simulink model "t1simu"  (R2023b)
settings: Solver=VariableStepAuto  StartTime=0.0  StopTime=10.0  RelTol=1e-3  EnableMultiTasking=on
settings Model: Creator=Admin  LastModifiedBy=danish
settings SolverCC: AlgebraicLoopSolver=TrustRegion
settings DataIOCC: ReturnWorkspaceOutputs=off
settings OptimizationCC: LifeSpan=inf
settings DebuggingCC: UnconnectedInputMsg=warning  UnconnectedOutputMsg=warning  UnconnectedLineMsg=warning  SFUnexpectedBacktrackingDiag=warning  SFNoUnconditionalDefaultTransitionDiag=warning  ArithmeticOperatorsInVariantConditions=warning
settings ModelReferenceCC: EnableRefExpFcnMdlSchedulingChecks=on
settings SFSimCC: SimUseLocalCustomCode=off  CustomCodeUndefinedFunction=UseInterfaceOnly
settings RTWCC: RTWUseLocalCustomCode=off
settings CodeAppCC: StateflowObjectComments=on
settings GRTTargetCC: TargetLangStandard=C89/C90 (ANSI)
settings ConfigComp: CovMetricSettings=dw  CovSaveCumulativeToWorkspaceVar=on  CovSaveSingleToWorkspaceVar=on  CovExternalEMLEnable=off

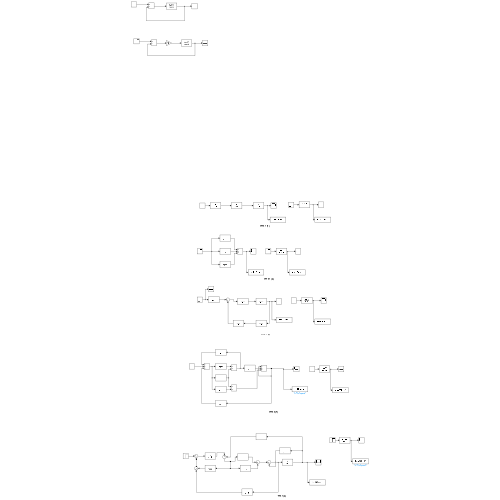
[thumbnail: Simulink's stored preview of the top-level diagram]
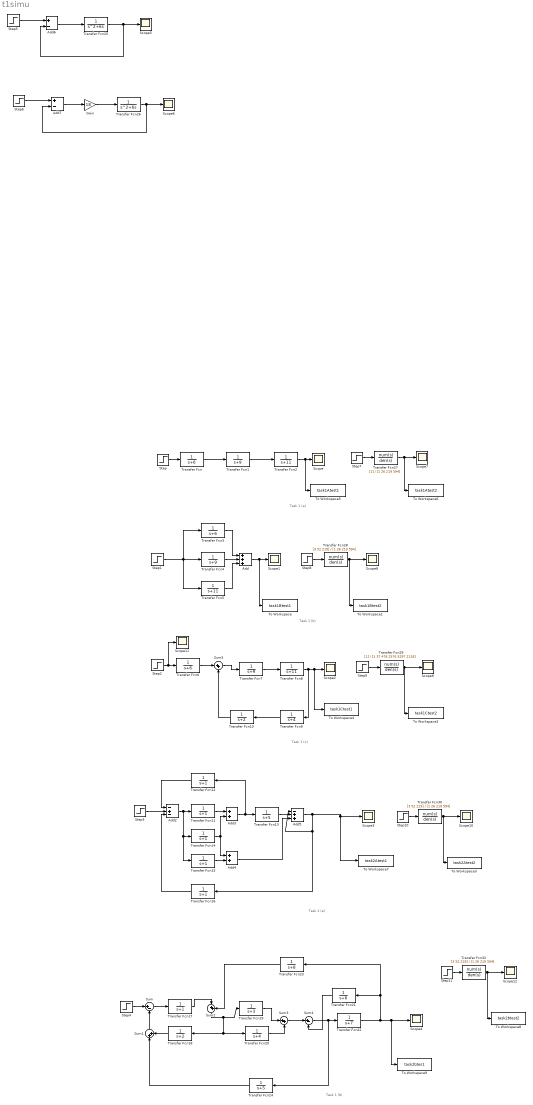
== system t1simu ==
  note: Task 1 (a)
  note: Task 1 (b)
  note: Task 1 (c)
  note: Task 2 (a)
  note: Task 1 (b)
  Add : Sum  Inputs=+++
  Add2 : Sum  Inputs=-+-
  Add3 : Sum
  Add4 : Sum
  Add5 : Sum  Inputs=-++
  Add6 : Sum  Inputs=+-
  Add7 : Sum  Inputs=+-
  Gain : Gain  Gain=18
  Scope{,1..12} (13 alike) : Scope
  Step{,1..11} (12 alike) : Step  Time=0  SampleTime=0
  Sum : Sum  Inputs=|+-
  Sum{1..3,5} (4 alike) : Sum  Inputs=|++
  Sum4 : Sum  Inputs=|+-
  To Workspace : ToWorkspace  VariableName=task1Btest1  SaveFormat=Timeseries  SampleTime=-1
  To Workspace1 : ToWorkspace  VariableName=task1Btest2  SaveFormat=Timeseries  SampleTime=-1
  To Workspace2 : ToWorkspace  VariableName=task1Ctest2  SaveFormat=Timeseries  SampleTime=-1
  To Workspace3 : ToWorkspace  VariableName=task2Atest2  SaveFormat=Timeseries  SampleTime=-1
  To Workspace4 : ToWorkspace  VariableName=task1Ctest1  SaveFormat=Timeseries  SampleTime=-1
  To Workspace5 : ToWorkspace  VariableName=task1Atest1  SaveFormat=Timeseries  SampleTime=-1
  To Workspace6 : ToWorkspace  VariableName=task1Atest2  SaveFormat=Timeseries  SampleTime=-1
  To Workspace7 : ToWorkspace  VariableName=task2Atest1  SaveFormat=Timeseries  SampleTime=-1
  To Workspace8 : ToWorkspace  VariableName=task2btest2  SaveFormat=Timeseries  SampleTime=-1
  To Workspace9 : ToWorkspace  VariableName=task2btes1  SaveFormat=Timeseries  SampleTime=-1
  Transfer Fcn{,3,6,21} (4 alike) : TransferFcn  Denominator=[1 6]
  Transfer Fcn1 : TransferFcn  Denominator=[1 9]
  Transfer Fcn10 : TransferFcn  Denominator=[1 2]
  Transfer Fcn{11..12,14..17} (6 alike) : TransferFcn  Denominator=[1 1]
  Transfer Fcn13 : TransferFcn  Denominator=[1 5]
  Transfer Fcn18 : TransferFcn  Denominator=[1 2]
  Transfer Fcn19 : TransferFcn  Denominator=[1 3]
  Transfer Fcn2 : TransferFcn  Denominator=[1 11]
  Transfer Fcn20 : TransferFcn  Denominator=[1 4]
  Transfer Fcn22 : TransferFcn  Denominator=[1 7]
  Transfer Fcn23 : TransferFcn  Denominator=[1 8]
  Transfer Fcn24 : TransferFcn  Denominator=[1 5]
  Transfer Fcn25 : TransferFcn  Denominator=[1 6 0]
  Transfer Fcn26 : TransferFcn  Denominator=[1 6 0]
  Transfer Fcn27 : TransferFcn  Denominator=[1 26 219 594]
  Transfer Fcn28 : TransferFcn  Numerator=[3 52 219]  Denominator=[1 26 219 594]
  Transfer Fcn29 : TransferFcn  Denominator=[1 37 478 2576 5297 2118]
  Transfer Fcn30 : TransferFcn  Numerator=[3 52 219]  Denominator=[1 26 219 594]
  Transfer Fcn32 : TransferFcn  Numerator=[3 52 219]  Denominator=[1 26 219 594]
  Transfer Fcn4 : TransferFcn  Denominator=[1 9]
  Transfer Fcn5 : TransferFcn  Denominator=[1 11]
  Transfer Fcn7 : TransferFcn  Denominator=[1 9]
  Transfer Fcn8 : TransferFcn  Denominator=[1 11]
  Transfer Fcn9 : TransferFcn  Denominator=[1 4]
  wires:
  Transfer Fcn1/1 -> Transfer Fcn2/1
  Transfer Fcn/1 -> Transfer Fcn1/1
  Step/1 -> Transfer Fcn/1
  Step1/1 -> Transfer Fcn3/1, Transfer Fcn5/1, Transfer Fcn4/1
  Transfer Fcn4/1 -> Add/2
  Transfer Fcn3/1 -> Add/1
  Transfer Fcn5/1 -> Add/3
  Add/1 -> To Workspace/1, Scope1/1
  Transfer Fcn6/1 -> Sum5/1
  Sum5/1 -> Transfer Fcn7/1
  Transfer Fcn7/1 -> Transfer Fcn8/1
  Transfer Fcn10/1 -> Sum5/2
  Transfer Fcn12/1 -> Add2/1
  Step3/1 -> Add2/2
  Transfer Fcn11/1 -> Add3/1
  Add2/1 -> Transfer Fcn15/1, Transfer Fcn14/1, Transfer Fcn11/1
  Add3/1 -> Transfer Fcn12/1, Transfer Fcn13/1
  Transfer Fcn14/1 -> Add4/1, Add3/2
  Transfer Fcn15/1 -> Add4/2
  Transfer Fcn13/1 -> Add5/2
  Transfer Fcn16/1 -> Add2/3
  Add4/1 -> Add5/3
  Step4/1 -> Sum/1
  Sum/1 -> Transfer Fcn17/1
  Sum1/1 -> Sum/2
  Transfer Fcn17/1 -> Sum2/1
  Transfer Fcn18/1 -> Sum1/2
  Sum2/1 -> Transfer Fcn20/1, Transfer Fcn18/1, Transfer Fcn19/1
  Transfer Fcn19/1 -> Sum3/1
  Transfer Fcn20/1 -> Sum3/2
  Sum3/1 -> Sum4/1
  Transfer Fcn21/1 -> Sum4/2
  Sum4/1 -> Transfer Fcn24/1, Transfer Fcn22/1
  Transfer Fcn22/1 -> Transfer Fcn23/1, Transfer Fcn21/1, Scope4/1, To Workspace9/1
  Transfer Fcn23/1 -> Sum2/2
  Transfer Fcn24/1 -> Sum1/1
  Add6/1 -> Transfer Fcn25/1
  Transfer Fcn25/1 -> Add6/2, Scope5/1
  Step5/1 -> Add6/1
  Step6/1 -> Add7/1
  Transfer Fcn26/1 -> Add7/2, Scope6/1
  Add7/1 -> Gain/1
  Gain/1 -> Transfer Fcn26/1
  Step7/1 -> Transfer Fcn27/1
  Step8/1 -> Transfer Fcn28/1
  Transfer Fcn28/1 -> To Workspace1/1, Scope8/1
  Transfer Fcn29/1 -> To Workspace2/1, Scope9/1
  Step9/1 -> Transfer Fcn29/1
  Transfer Fcn30/1 -> To Workspace3/1, Scope10/1
  Step10/1 -> Transfer Fcn30/1
  Add5/1 -> To Workspace7/1, Scope3/1, Add5/1, Transfer Fcn16/1
  Step2/1 -> Scope11/1, Transfer Fcn6/1
  Transfer Fcn8/1 -> Transfer Fcn9/1, To Workspace4/1, Scope2/1
  Transfer Fcn2/1 -> To Workspace5/1, Scope/1
  Transfer Fcn27/1 -> To Workspace6/1, Scope7/1
  Transfer Fcn9/1 -> Transfer Fcn10/1
  Step11/1 -> Transfer Fcn32/1
  Transfer Fcn32/1 -> To Workspace8/1, Scope12/1
